simulink model "sm_bread_slicer"  (R2021b)
settings: Solver=ode15s  StartTime=0.0  StopTime=10  MaxStep=0.01  RelTol=1e-3  EnableMultiTasking=on
model workspace (MATLAB code in the model file):
  | lgrey = [0.6 0.6 0.6];
  | dgrey = [0.4 0.4 0.4];
  | blue = [0.0 0.6 1.0];
  | orange = [0.8 0.5 0.0];
  | dgreen = [0.0 0.3 0.0];
  | brown = [0.3 0.2 0.0];
  | red = [0.9 0.3 0.2];
  | yellow = [0.9 0.7 0.2];
  | rho_alum = 2700;
undefined symbols (not defined in the file): X, Y, Z
libraries: sm_lib x22, sm_bread_slicer_lib x10, fl_lib x8, nesl_utility x1
Description:
  | Rotational Interface : Electrically Operated Bread Slicer
  | 
  | This model simulates an electrically operated 1-DOF bread
  | slicing mechanism. The electrical motor circuit is modeled in
  | Simscape(TM) while the bread slicing mechanism is modeled
  | in Simscape Multibody(TM). The model uses a Revolute-Rotational
  | Interface block (blue block) to interface the electrical and 3D
  | mechanical parts of the model.
settings Model: Creator=The MathWorks, Inc.  LastModifiedBy=The MathWorks, Inc.
settings SolverCC: AlgebraicLoopSolver=TrustRegion
settings DataIOCC: LimitDataPoints=on  SaveFormat=Array  ReturnWorkspaceOutputs=off
settings OptimizationCC: ExpressionDepthLimit=2147483647  LifeSpan=inf
settings DebuggingCC: UnderspecifiedInitializationDetection=Classic  MergeDetectMultiDrivingBlocksExec=none  SolverPrmCheckMsg=warning  StateNameClashWarn=warning  SFUnexpectedBacktrackingDiag=warning  SFNoUnconditionalDefaultTransitionDiag=warning  SFExecutionAtInitializationDiag=none  SFMachineParentedDataDiag=warning  ArithmeticOperatorsInVariantConditions=warning
settings HardwareCC: ProdBitPerPointer=32  ProdBitPerSizeT=32  ProdBitPerPtrDiffT=32  ProdLargestAtomicFloat=None  ProdIntDivRoundTo=Undefined  ProdEndianess=Unspecified  ProdWordSize=32  ProdHWDeviceType=32-bit Generic
settings ModelReferenceCC: PropagateSignalLabelsOutOfModel=off
settings SFSimCC: SimUseLocalCustomCode=off  CustomCodeUndefinedFunction=UseInterfaceOnly
settings RTWCC: RTWUseLocalCustomCode=off
settings CodeAppCC: StateflowObjectComments=on
settings GRTTargetCC: TargetLangStandard=C89/C90 (ANSI)
settings ConfigComp: CovMetricSettings=dw  CovSaveCumulativeToWorkspaceVar=on  CovSaveSingleToWorkspaceVar=on  CovExternalEMLEnable=off  CovSFcnEnable=off
settings SimscapeCC: SimscapeNormalizeSystem=off  SimscapeLogType=all  SimscapeLogSimulationStatistics=on  SimscapeLogName=simlog_sm_bread_slicer
settings ConfigurationSet: Description=SimMechanics 2G
settings DiagnosticsConfigSet: SimMechanicsUnconnectedFramePorts=none
settings ExplorerConfigSet: InternalSimMechanicsExplorerSettings="<ExplorerConfiguration><canonicalview>default</canonicalview><TilePanel><TileInfo><Tiles Columns=\"1\" Count=\"1\" Rows=\"1\"><Column Left=\"2\" Weight=\"1\"/><Column Left=\"418\"/><Row Top=\"2\" Weight=\"1\"/><Row Top=\"419\"/><Tile Height=\"1\" Width=\"1\" X=\"0\" Y=\"0\"/></Tiles></TileInfo><SceneInfo><SceneViewer><BGColor><R>0.60000002384185791</R><G>0.60000002384185791</G><B>0.60000002384185791</B></BGColor><Camera><Position><X>0.97822830794307525</X><Y>-0.8448557030961209</Y><Z>0.99010983822795684</Z></Position><Center><X>0.13337260484695435</X><Y>0</Y><Z>0.14525413513183594</Z></Center><Up><X>-0.40824829046386307</X><Y>0.40824829046386307</Y><Z>0.81649658092772615</Z></Up><Left>-0.49494555294513704</Left><Right>0.49494555294513704</Right><Bottom>-0.45368637889623642</Bottom><Top>0.45368637889623642</Top></Camera></SceneViewer></SceneInfo></TilePanel></ExplorerConfiguration>"

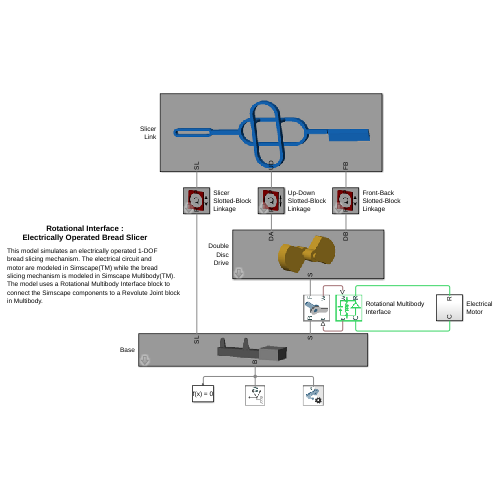
[thumbnail: Simulink's stored preview of the top-level diagram]
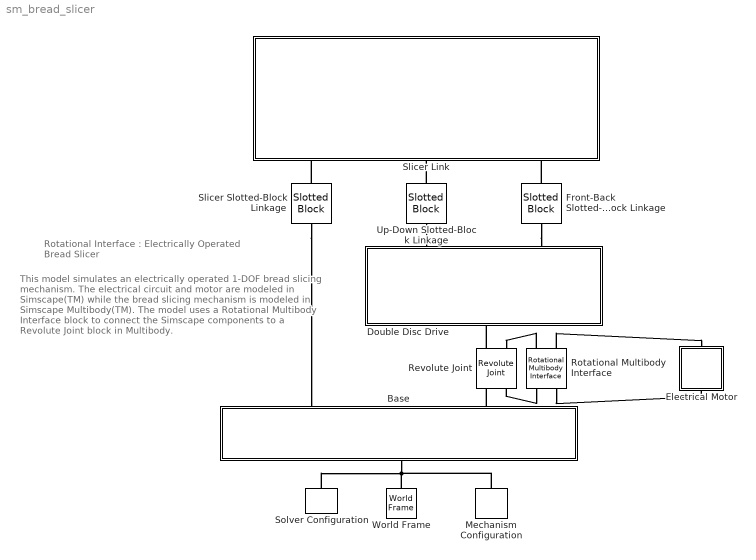
== system sm_bread_slicer ==
  note: This model simulates an electrically operated 1-DOF
      | bread slicing mechanism. The electrical circuit and
      | motor are modeled in Simscape(TM) while the bread
      | slicing mechanism is modeled in Simscape Multibody(TM).
      | The model uses a Rotational Multibody Interface block to
      | connect the Simscape components to a Revolute Joint block in Multibody.
  note: Rotational Interface :
      | Electrically Operated Bread Slicer
  Base : Subsystem  mask(Bread Slicer Base){L=70, W=15, H=10, Lct=30, Wct=30, Hct=14, Oha=-30, Ha=12, Wa=8, Ta=2, Rta=3, Rpa=0.75, Lpa=9, Hb=15, Wb=12, Tb=1.5, Rtb=3, clr=dgrey, rho=rho_alum}
      mask prompts: L "Base length (cm):"; W "Base width (cm):"; H "Base height (cm):"; Lct "Cutting table length (cm):"; Wct "Cutting table width (cm):"; Hct "Cutting table height (cm):"; Oha "Offset (cm):"; Ha "Height of hinge (cm):"; Wa "Base width of hinge (cm):"; Ta "Thickness of hinge (cm):"; Rta "Radius of curvature of top (cm):"; Rpa "Radius of pin:"; Lpa "Length of pin:"; Hb "Height of hinge (cm):"; Wb "Base width of hinge (cm):"; Tb "Thickness of hinge (cm):"; Rtb "Radius of curvature of top (cm):"; clr "Color:"; rho "Density (kg/m^3):"
      mask help: Base ground body on which the bread slicer mechanism is mounted on.
      mask Display:
      | image('sm_bread_slicer_base.png');
      | port_label('RConn',1,'SL');
      | port_label('RConn',2,'S');
      | port_label('LConn',1,'B');
  Double Disc Drive : Subsystem  mask(Double Disc Drive){R=5, T=4, Sa=150, S=6, Op=3, Rp=1, Lp=12, clr=yellow, rho=rho_alum}
      mask prompts: R "Disc radius (cm):"; T "Disc thickness (cm):"; Sa "Disc sector angle (deg):"; S "Disc separation (cm):"; Op "Pin offset (cm):"; Rp "Pin radius (cm):"; Lp "Pin length (cm):"; clr "Disc color [r g b]:"; rho "Density (kg/m^3):"
      mask help: Shaft with two rigidly attached opposing disc segments. The disc segments can fit and revolve within circular cavities. The port S refers to the shaft frame and must be attached to a revolute joint. The ports DA and DB refer to the frames at the center of the disc segments.
      mask init:
      | Sar = Sa*pi/180;
      | theta = linspace(-Sar/2,Sar/2,100)';
      | disc_xsec = [R*cos(theta) R*sin(theta)];
      | theta = linspace(Sar/2,2*pi-Sar/2,200)';
      | disc_xsec = [disc_xsec; 2*Rp*cos(theta)-Op 2*Rp*sin(theta)];
      mask Display:
      | image('sm_bread_slicer_drive.png');
      | port_label('RConn',1,'DA');
      | port_label('RConn',2,'DB');
      | port_label('LConn',1,'S');
  Electrical Motor : Subsystem
  Front-Back Slotted-Block Linkage : sm_bread_slicer_lib/Slotted Block  Lb=12  Wb=11  Tb=2  Rh=5  clr=red  rho=rho_alum
      settings: SourceProductBaseCode=MS
  Mechanism Configuration : sm_lib/Utilities/Mechanism Configuration  UniformGravity=Constant  GravityVector=[0 0 -9.81]  GravityUnits=m/s^2  LinearizationDelta=0.001  JointModeTransitionNonlinearIterations=2
  Revolute Joint : sm_lib/Joints/Revolute Joint  JointMode=Normal  SenseConstraintForce=off  SenseConstraintForceX=off  SenseConstraintForceY=off  SenseConstraintForceZ=off  SenseConstraintTorque=off  SenseConstraintTorqueX=off  SenseConstraintTorqueY=off  SenseConstraintTorqueZ=off  SenseTotalForce=off  SenseTotalForceX=off  SenseTotalForceY=off  SenseTotalForceZ=off  SenseTotalTorque=off  SenseTotalTorqueX=off  SenseTotalTorqueY=off  SenseTotalTorqueZ=off  CompositeWrenchDir=FollowerOnBase  CompositeWrenchFrame=BaseFrame  EquilibriumPosition=0  EquilibriumPositionUnits=deg  SpringStiffness=0  SpringStiffnessUnits=N*m/deg  DampingCoefficient=0  DampingCoefficientUnits=N*m/(deg/s)  TorqueActuationMode=InputTorque  MotionActuationMode=ComputedMotion  SensePosition=off  SenseVelocity=on  SenseAcceleration=off  SenseTorqueForce=off  SenseLowerLimitTorqueForce=off  SenseUpperLimitTorqueForce=off  LowerLimitSpecify=off  LowerLimitBound=-90  LowerLimitBoundUnits=deg  LowerLimitStiffness=1e4  LowerLimitStiffnessUnits=N*m/deg  LowerLimitDamping=10  LowerLimitDampingUnits=N*m/(deg/s)  LowerLimitTransitionRegionWidth=0.1  LowerLimitTransitionRegionWidthUnits=deg  UpperLimitSpecify=off  UpperLimitBound=90  UpperLimitBoundUnits=deg  UpperLimitStiffness=1e4  UpperLimitStiffnessUnits=N*m/deg  UpperLimitDamping=10  UpperLimitDampingUnits=N*m/(deg/s)  UpperLimitTransitionRegionWidth=0.1  UpperLimitTransitionRegionWidthUnits=deg  PositionTargetSpecify=on  PositionTargetPriority=Low  PositionTargetValue=90  PositionTargetValueUnits=deg  VelocityTargetSpecify=off  VelocityTargetPriority=High  VelocityTargetValue=0  VelocityTargetValueUnits=deg/s
  Rotational Multibody Interface : fl_lib/Mechanical/Multibody Interfaces/Rotational Multibody Interface
      settings: SourceProductBaseCode=SS
  Slicer Link : Subsystem  mask(Bread Slicer Link){}
      mask Display:
      | image('sm_bread_slicer_link.png');
      | port_label('LConn',1,'SL');
      | port_label('LConn',2,'UD');
      | port_label('LConn',3,'FB');
  Slicer Slotted-Block Linkage : sm_bread_slicer_lib/Slotted Block  Lb=4  Wb=2  Tb=2  Rh=0.75  clr=red  rho=rho_alum
      settings: SourceProductBaseCode=MS
  Solver Configuration : nesl_utility/Solver Configuration  PhysicalDomain=network_engine_domain  SubClassName=solver  LeftPortType=input  RightPortType=generic  Tones=[]  Harmonics=[]  SimulateNoise=off  Profile=off  UseLocalSampling=off  EnableSwitchedLinearOptims=on  FrequencyDomain=off  UseCCode=off  RelTol=0.001  AbsTol=1e-06  MinStep=1e-09  ToWorkspace=off  RevertToSquareIcSolve=off  NumHomotopyIterations=100  PhasorMode=off  PhasorModeNumHarmonics=1  DoDC=off  ResidualTolerance=1e-9  UseLocalSolver=off  LocalSolverChoice=NE_BACKWARD_EULER_ADVANCER  LocalSolverSampleTime=.001  DoFixedCost=off  MaxNonlinIter=3  MaxModeIter=2  ComputeImpulses=off  ImpulseIterations=2  LinearAlgebra=Sparse  EquationFormulation=NE_TIME_EF  DelaysMemoryBudget=1024  AutomaticFiltering=on  FilteringTimeConstant=0.001  PartitionStorageMethod=AS_NEEDED  PartitionMemoryBudget=1024  PartitionMethod=FAST
      settings: SourceProductBaseCode=PW,SS
  Up-Down Slotted-Block Linkage : sm_bread_slicer_lib/Slotted Block  Lb=12  Wb=11  Tb=2  Rh=5  clr=red  rho=rho_alum
      settings: SourceProductBaseCode=MS
  World Frame : sm_lib/Frames and Transforms/World Frame
  connections:
  World Frame/RConn1 -- Mechanism Configuration/RConn1 -- Solver Configuration/RConn1 -- Base/LConn1
  Slicer Slotted-Block Linkage/RConn1 -- Slicer Link/LConn1
  Slicer Slotted-Block Linkage/LConn1 -- Base/RConn1
  Up-Down Slotted-Block Linkage/RConn1 -- Slicer Link/LConn2
  Up-Down Slotted-Block Linkage/LConn1 -- Double Disc Drive/RConn1
  Front-Back Slotted-Block Linkage/RConn1 -- Slicer Link/LConn3
  Front-Back Slotted-Block Linkage/LConn1 -- Double Disc Drive/RConn2
  Revolute Joint/RConn1 -- Double Disc Drive/LConn1
  Rotational Multibody Interface/RConn1 -- Revolute Joint/RConn2
  Rotational Multibody Interface/LConn1 -- Revolute Joint/LConn2
  Base/RConn2 -- Revolute Joint/LConn1
  Rotational Multibody Interface/LConn2 -- Electrical Motor/LConn1
  Rotational Multibody Interface/RConn2 -- Electrical Motor/RConn1

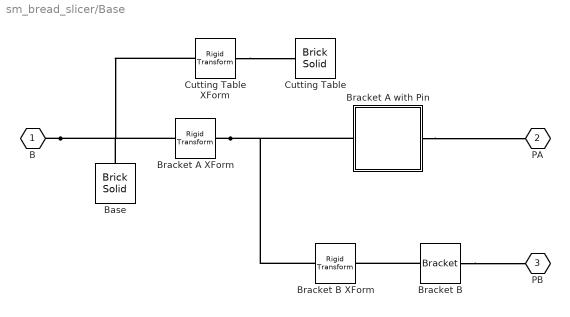
== system sm_bread_slicer/Base ==
  Base : sm_lib/Body Elements/Brick Solid  GraphicAmbientColor=[0.15 0.15 0.15 1.0]  BasedOnType=Density  BrickDimensions=[L W H]  BrickDimensionUnits=cm  CenterOfMass=[0 0 0]  CenterOfMassUnits=m  GraphicDiffuseColor=clr  Density=1000  DensityUnits=kg/(m^3)  DoExposeReferenceFrame=on  GraphicEmissiveColor=[0.0 0.0 0.0 1.0]  ExportEntireGeometry=off  SerializedFrames=<Frames/>  MarkerShape=Sphere  MarkerSize=10  GraphicType=FromGeometry  InertiaType=CalculateFromGeometry  Mass=1  MassUnits=kg  MomentsOfInertia=[1 1 1]  MomentsOfInertiaUnits=kg*m^2  GraphicOpacity=1.0  ProductsOfInertia=[0 0 0]  ProductsOfInertiaUnits=kg*m^2  GraphicShininess=75  GraphicSpecularColor=[0.5 0.5 0.5 1.0]  GraphicVisPropType=SimpleVisualProperties
  Bracket A XForm : sm_lib/Frames and Transforms/Rigid Transform  TranslationMethod=Cartesian  TranslationStandardOffset=0  TranslationLengthUnit=cm  TranslationStandardAxis=+Z  TranslationCartesianOffset=[Oha 0 H/2]  TranslationROffset=0  TranslationROffsetUnits=m  TranslationZOffset=0  TranslationZOffsetUnits=m  TranslationThetaOffset=0  TranslationThetaOffsetUnits=deg  RotationMethod=AlignedAxes  RotationAngleUnits=deg  RotationStandardAxis=+Z  RotationAngle=0  RotationArbitraryAxis=[0 0 1]  FollAlignAxisA=+Y  BaseAlignAxisA=+Z  FollAlignAxisB=+Z  BaseAlignAxisB=-Y  RotationSequenceAxes=FollowerAxes  RotationSequence=XYX  RotationSequenceAngles=[0 0 0]  RotationSequenceAnglesUnits=deg  RotationMatrix=[1 0 0; 0 1 0; 0 0 1]
  Bracket A with Pin : Subsystem  mask(Bracket with Pin){H=Ha, W=Wa, T=Ta, Rt=Rta, Rp=Rpa, Lp=Lpa, Oh=3, clr=clr, rho=rho}
      mask prompts: H "Height of hinge (cm):"; W "Base width of hinge (cm):"; T "Thickness of hinge (cm):"; Rt "Radius of curvature of top (cm):"; Rp "Pin radius (cm):"; Lp "Pin length (cm):"; Oh "Hinge point offset (cm)"; clr "Color:"; rho "Density:"
      mask init:
      | d = sqrt((H-Rt)^2 + (W/2)^2);
      | thd = acos(Rt/d) + acos((H-Rt)/d) - pi/2;
      | theta = linspace(thd,pi-thd,100)';
      | hinge_xsec = [W/2 0; Rt*cos(theta) (H-Rt)+Rt*sin(theta); -W/2 0];
  Bracket B : sm_bread_slicer_lib/Bracket  H=Hb  W=Wb  T=Tb  Rt=Rtb  clr=clr  rho=rho
      settings: SourceProductBaseCode=MS
  Bracket B XForm : sm_lib/Frames and Transforms/Rigid Transform  TranslationMethod=Cartesian  TranslationStandardOffset=39.5  TranslationLengthUnit=cm  TranslationStandardAxis=+X  TranslationCartesianOffset=[39.5 0 6]  TranslationROffset=0  TranslationROffsetUnits=m  TranslationZOffset=0  TranslationZOffsetUnits=m  TranslationThetaOffset=0  TranslationThetaOffsetUnits=deg  RotationMethod=None  RotationAngleUnits=deg  RotationStandardAxis=+Z  RotationAngle=90  RotationArbitraryAxis=[0 0 1]  FollAlignAxisA=+X  BaseAlignAxisA=+Y  FollAlignAxisB=+Y  BaseAlignAxisB=+Z  RotationSequenceAxes=FollowerAxes  RotationSequence=XYX  RotationSequenceAngles=[0 0 0]  RotationSequenceAnglesUnits=deg  RotationMatrix=[1 0 0; 0 1 0; 0 0 1]
  Cutting Table : sm_lib/Body Elements/Brick Solid  GraphicAmbientColor=[0.15 0.15 0.15 1.0]  BasedOnType=Density  BrickDimensions=[Lct Wct Hct]  BrickDimensionUnits=cm  CenterOfMass=[0 0 0]  CenterOfMassUnits=m  GraphicDiffuseColor=clr+0.2  Density=1000  DensityUnits=kg/(m^3)  DoExposeReferenceFrame=on  GraphicEmissiveColor=[0.0 0.0 0.0 1.0]  ExportEntireGeometry=off  SerializedFrames=<Frames/>  MarkerShape=Sphere  MarkerSize=10  GraphicType=FromGeometry  InertiaType=CalculateFromGeometry  Mass=1  MassUnits=kg  MomentsOfInertia=[1 1 1]  MomentsOfInertiaUnits=kg*m^2  GraphicOpacity=1.0  ProductsOfInertia=[0 0 0]  ProductsOfInertiaUnits=kg*m^2  GraphicShininess=75  GraphicSpecularColor=[0.5 0.5 0.5 1.0]  GraphicVisPropType=SimpleVisualProperties
  Cutting Table XForm : sm_lib/Frames and Transforms/Rigid Transform  TranslationMethod=Cartesian  TranslationStandardOffset=0  TranslationLengthUnit=cm  TranslationStandardAxis=+X  TranslationCartesianOffset=[L/2+Lct/2 0 (Hct-H)/2]  TranslationROffset=0  TranslationROffsetUnits=m  TranslationZOffset=0  TranslationZOffsetUnits=m  TranslationThetaOffset=0  TranslationThetaOffsetUnits=deg  RotationMethod=None  RotationAngleUnits=deg  RotationStandardAxis=+Z  RotationAngle=0  RotationArbitraryAxis=[0 0 1]  FollAlignAxisA=+Y  BaseAlignAxisA=+Z  FollAlignAxisB=+Z  BaseAlignAxisB=-Y  RotationSequenceAxes=FollowerAxes  RotationSequence=XYX  RotationSequenceAngles=[0 0 0]  RotationSequenceAnglesUnits=deg  RotationMatrix=[1 0 0; 0 1 0; 0 0 1]
  B : PMIOPort  Side=Left
  PA : PMIOPort  Port=2  Side=Right
  PB : PMIOPort  Port=3  Side=Right
  connections:
  B/RConn1 -- Base/RConn1 -- Cutting Table XForm/LConn1 -- Bracket A XForm/LConn1
  Bracket A XForm/RConn1 -- Bracket B XForm/LConn1 -- Bracket A with Pin/LConn1
  Bracket B/RConn1 -- PB/RConn1
  Cutting Table XForm/RConn1 -- Cutting Table/RConn1
  Bracket B/LConn1 -- Bracket B XForm/RConn1
  Bracket A with Pin/RConn1 -- PA/RConn1

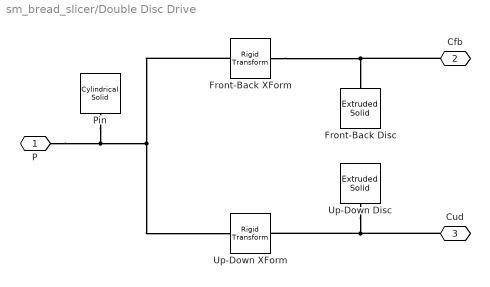
== system sm_bread_slicer/Double Disc Drive ==
  Front-Back Disc : sm_lib/Body Elements/Extruded Solid  GraphicAmbientColor=[0.15 0.15 0.15 1.0]  BasedOnType=Density  CenterOfMass=[0 0 0]  CenterOfMassUnits=m  GraphicDiffuseColor=clr  ExportConvexHullGeometry=off  ExtrusionCrossSection=disc_xsec  ExtrusionCrossSectionUnits=cm  Density=rho  DensityUnits=kg/(m^3)  DoExposeReferenceFrame=on  GraphicEmissiveColor=[0.0 0.0 0.0 1.0]  ExportEntireGeometry=off  ExtrusionLength=T  ExtrusionLengthUnits=cm  ExtrusionType=General  SerializedFrames=<Frames/>  MarkerShape=Sphere  MarkerSize=10  GraphicType=FromGeometry  InertiaType=CalculateFromGeometry  Mass=1  MassUnits=kg  MomentsOfInertia=[1 1 1]  MomentsOfInertiaUnits=kg*m^2  PolygonNumSides=3  GraphicOpacity=1.0  PolygonOuterRadius=1  PolygonOuterRadiusUnits=m  ProductsOfInertia=[0 0 0]  ProductsOfInertiaUnits=kg*m^2  GraphicShininess=75  GraphicSpecularColor=[0.5 0.5 0.5 1.0]  GraphicVisPropType=SimpleVisualProperties
  Front-Back XForm : sm_lib/Frames and Transforms/Rigid Transform  TranslationMethod=Cartesian  TranslationStandardOffset=0  TranslationLengthUnit=cm  TranslationStandardAxis=+Y  TranslationCartesianOffset=[-Op 0 -S/2]  TranslationROffset=0  TranslationROffsetUnits=m  TranslationZOffset=0  TranslationZOffsetUnits=m  TranslationThetaOffset=0  TranslationThetaOffsetUnits=deg  RotationMethod=AlignedAxes  RotationAngleUnits=deg  RotationStandardAxis=+Z  RotationAngle=90  RotationArbitraryAxis=[0 0 1]  FollAlignAxisA=+X  BaseAlignAxisA=-X  FollAlignAxisB=+Y  BaseAlignAxisB=-Y  RotationSequenceAxes=FollowerAxes  RotationSequence=XYX  RotationSequenceAngles=[0 0 0]  RotationSequenceAnglesUnits=deg  RotationMatrix=[1 0 0; 0 1 0; 0 0 1]
  Pin : sm_lib/Body Elements/Cylindrical Solid  GraphicAmbientColor=[0.15 0.15 0.15 1.0]  BasedOnType=Density  CenterOfMass=[0 0 0]  CenterOfMassUnits=m  GraphicDiffuseColor=clr  CylinderLength=Lp  CylinderLengthUnits=cm  CylinderRadius=Rp  CylinderRadiusUnits=cm  Density=rho  DensityUnits=kg/(m^3)  DoExposeReferenceFrame=on  GraphicEmissiveColor=[0.0 0.0 0.0 1.0]  ExportEntireGeometry=off  SerializedFrames=<Frames/>  MarkerShape=Sphere  MarkerSize=10  GraphicType=FromGeometry  InertiaType=CalculateFromGeometry  Mass=1  MassUnits=kg  MomentsOfInertia=[1 1 1]  MomentsOfInertiaUnits=kg*m^2  GraphicOpacity=1.0  ProductsOfInertia=[0 0 0]  ProductsOfInertiaUnits=kg*m^2  GraphicShininess=75  GraphicSpecularColor=[0.5 0.5 0.5 1.0]  GraphicVisPropType=SimpleVisualProperties
  Up-Down Disc : sm_lib/Body Elements/Extruded Solid  GraphicAmbientColor=[0.15 0.15 0.15 1.0]  BasedOnType=Density  CenterOfMass=[0 0 0]  CenterOfMassUnits=m  GraphicDiffuseColor=clr  ExportConvexHullGeometry=off  ExtrusionCrossSection=disc_xsec  ExtrusionCrossSectionUnits=cm  Density=rho  DensityUnits=kg/(m^3)  DoExposeReferenceFrame=on  GraphicEmissiveColor=[0.0 0.0 0.0 1.0]  ExportEntireGeometry=off  ExtrusionLength=T  ExtrusionLengthUnits=cm  ExtrusionType=General  SerializedFrames=<Frames/>  MarkerShape=Sphere  MarkerSize=10  GraphicType=FromGeometry  InertiaType=CalculateFromGeometry  Mass=1  MassUnits=kg  MomentsOfInertia=[1 1 1]  MomentsOfInertiaUnits=kg*m^2  PolygonNumSides=3  GraphicOpacity=1.0  PolygonOuterRadius=1  PolygonOuterRadiusUnits=m  ProductsOfInertia=[0 0 0]  ProductsOfInertiaUnits=kg*m^2  GraphicShininess=75  GraphicSpecularColor=[0.5 0.5 0.5 1.0]  GraphicVisPropType=SimpleVisualProperties
  Up-Down XForm : sm_lib/Frames and Transforms/Rigid Transform  TranslationMethod=Cartesian  TranslationStandardOffset=0  TranslationLengthUnit=cm  TranslationStandardAxis=-Y  TranslationCartesianOffset=[Op 0 S/2]  TranslationROffset=0  TranslationROffsetUnits=m  TranslationZOffset=0  TranslationZOffsetUnits=m  TranslationThetaOffset=0  TranslationThetaOffsetUnits=deg  RotationMethod=None  RotationAngleUnits=deg  RotationStandardAxis=+Z  RotationAngle=90  RotationArbitraryAxis=[0 0 1]  FollAlignAxisA=+X  BaseAlignAxisA=+Y  FollAlignAxisB=+Y  BaseAlignAxisB=-X  RotationSequenceAxes=FollowerAxes  RotationSequence=XYX  RotationSequenceAngles=[0 0 0]  RotationSequenceAnglesUnits=deg  RotationMatrix=[1 0 0; 0 1 0; 0 0 1]
  P : PMIOPort  Side=Left
  Cfb : PMIOPort  Port=2  Side=Right
  Cud : PMIOPort  Port=3  Side=Right
  connections:
  Up-Down Disc/RConn1 -- Cud/RConn1 -- Up-Down XForm/RConn1
  Pin/RConn1 -- P/RConn1 -- Front-Back XForm/LConn1 -- Up-Down XForm/LConn1
  Front-Back XForm/RConn1 -- Cfb/RConn1 -- Front-Back Disc/RConn1

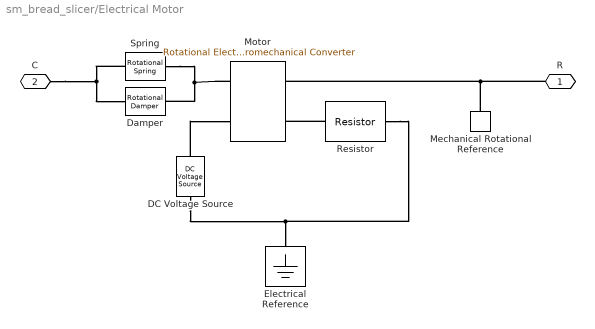
== system sm_bread_slicer/Electrical Motor ==
  DC Voltage Source : fl_lib/Electrical/Electrical Sources/DC Voltage Source  v0=50 V
  Damper : fl_lib/Mechanical/Rotational Elements/Rotational Damper  D=0.001 N*m/(rad/s)  w_specify=off  w_priority=High  w=0 rad/s  w_nominal_specify=off  w_nominal_unit=rad/s  w_nominal_value=1  t_specify=off  t_priority=High  t=0 N*m  t_nominal_specify=off  t_nominal_unit=N*m  t_nominal_value=1
  Electrical Reference : fl_lib/Electrical/Electrical Elements/Electrical Reference
  Mechanical Rotational Reference : fl_lib/Mechanical/Rotational Elements/Mechanical Rotational Reference
  Motor : fl_lib/Electrical/Electrical Elements/Rotational Electromechanical Converter  K=-5 V/(rad/s)  i_specify=off  i_priority=High  i=0 A  i_nominal_specify=off  i_nominal_unit=A  i_nominal_value=1  v_specify=off  v_priority=High  v=0 V  v_nominal_specify=off  v_nominal_unit=V  v_nominal_value=1  t_specify=off  t_priority=High  t=0 N*m  t_nominal_specify=off  t_nominal_unit=N*m  t_nominal_value=1  w_specify=off  w_priority=High  w=0 rad/s  w_nominal_specify=off  w_nominal_unit=rad/s  w_nominal_value=1
  Resistor : fl_lib/Electrical/Electrical Elements/Resistor  R=1 Ohm  i_specify=off  i_priority=High  i=0 A  i_nominal_specify=off  i_nominal_unit=A  i_nominal_value=1  v_specify=off  v_priority=High  v=0 V  v_nominal_specify=off  v_nominal_unit=V  v_nominal_value=1
  Spring : fl_lib/Mechanical/Rotational Elements/Rotational Spring  spr_rate=10 N*m/rad  w_specify=off  w_priority=High  w=0 rad/s  w_nominal_specify=off  w_nominal_unit=rad/s  w_nominal_value=1  t_specify=off  t_priority=High  t=0 N*m  t_nominal_specify=off  t_nominal_unit=N*m  t_nominal_value=1  phi_specify=on  phi_priority=High  phi=0 rad  phi_nominal_specify=off  phi_nominal_unit=rad  phi_nominal_value=1
  R : PMIOPort  Side=Right
  C : PMIOPort  Port=2  Side=Left
  connections:
  Spring/LConn1 -- C/RConn1 -- Damper/LConn1
  Spring/RConn1 -- Motor/LConn2 -- Damper/RConn1
  DC Voltage Source/LConn1 -- Motor/LConn1
  Resistor/LConn1 -- Motor/RConn1
  DC Voltage Source/RConn1 -- Electrical Reference/LConn1 -- Resistor/RConn1
  R/RConn1 -- Mechanical Rotational Reference/LConn1 -- Motor/RConn2

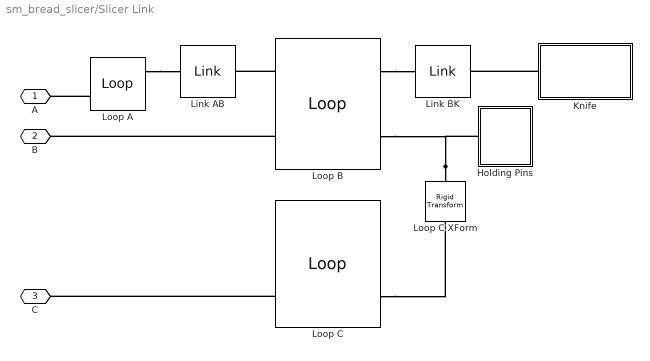
== system sm_bread_slicer/Slicer Link ==
  Holding Pins : Subsystem
  Knife : Subsystem  mask{L=20, W=6, Wb=2, Tb=0.5, clr=blue, rho=rho_alum}
      mask prompts: L "Length of knife (cm):"; W "Total width of knife (cm):"; Wb "Base width of knife (cm):"; Tb "Base thickness of knife (cm):"; clr "Color [r g b]:"; rho "Density (kg/m^3):"
      mask init:
      | knife_xsec = [0 -Tb/2; Wb -Tb/2; W 0; Wb Tb/2; 0 Tb/2];
      mask Display: image('sm_bread_slicer_knife.png');
  Link AB : sm_bread_slicer_lib/Link  L=11  W=2  T=2  Rl=2  Rr=7  clr=blue  rho=rho_alum
      settings: SourceProductBaseCode=MS
  Link BK : sm_bread_slicer_lib/Link  L=10  W=2  T=2  Rl=7  Rr=1000  clr=blue  rho=rho_alum
      settings: SourceProductBaseCode=MS
  Loop A : sm_bread_slicer_lib/Loop  L=15  W=4  T=2  Ws=2  clr=blue  rho=rho_alum
      settings: SourceProductBaseCode=MS
  Loop B : sm_bread_slicer_lib/Loop  L=25  W=14  T=2  Ws=11  clr=blue  rho=rho_alum
      settings: SourceProductBaseCode=MS
  Loop C : sm_bread_slicer_lib/Loop  L=25  W=14  T=2  Ws=11  clr=blue  rho=rho_alum
      settings: SourceProductBaseCode=MS
  Loop C XForm : sm_lib/Frames and Transforms/Rigid Transform  TranslationMethod=Cartesian  TranslationStandardOffset=6  TranslationLengthUnit=cm  TranslationStandardAxis=+Z  TranslationCartesianOffset=[0 0 6]  TranslationROffset=0  TranslationROffsetUnits=m  TranslationZOffset=0  TranslationZOffsetUnits=m  TranslationThetaOffset=0  TranslationThetaOffsetUnits=deg  RotationMethod=StandardAxis  RotationAngleUnits=deg  RotationStandardAxis=+Z  RotationAngle=90  RotationArbitraryAxis=[0 0 1]  FollAlignAxisA=+X  BaseAlignAxisA=+Y  FollAlignAxisB=+Y  BaseAlignAxisB=+Z  RotationSequenceAxes=FollowerAxes  RotationSequence=XYX  RotationSequenceAngles=[0 0 0]  RotationSequenceAnglesUnits=deg  RotationMatrix=[1 0 0; 0 1 0; 0 0 1]
  A : PMIOPort  Side=Left
  B : PMIOPort  Port=2  Side=Left
  C : PMIOPort  Port=3  Side=Left
  connections:
  Loop A/RConn1 -- Link AB/LConn1
  Loop A/LConn2 -- A/RConn1
  Loop B/LConn1 -- Link AB/RConn1
  Loop B/RConn1 -- Link BK/LConn1
  Loop C XForm/LConn1 -- Holding Pins/LConn1 -- Loop B/RConn2
  Loop C/RConn2 -- Loop C XForm/RConn1
  Loop C/LConn2 -- C/RConn1
  Loop B/LConn2 -- B/RConn1
  Knife/LConn1 -- Link BK/RConn1

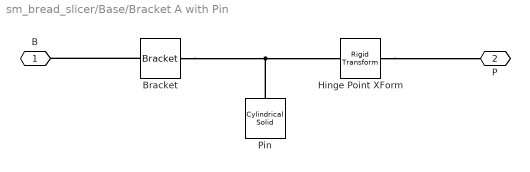
== system sm_bread_slicer/Base/Bracket A with Pin ==
  Bracket : sm_bread_slicer_lib/Bracket  H=H  W=W  T=T  Rt=Rt  clr=clr  rho=rho
      settings: SourceProductBaseCode=MS
  Hinge Point XForm : sm_lib/Frames and Transforms/Rigid Transform  TranslationMethod=Cartesian  TranslationStandardOffset=0  TranslationLengthUnit=cm  TranslationStandardAxis=+Y  TranslationCartesianOffset=[0 0 Oh]  TranslationROffset=0  TranslationROffsetUnits=m  TranslationZOffset=0  TranslationZOffsetUnits=m  TranslationThetaOffset=0  TranslationThetaOffsetUnits=deg  RotationMethod=None  RotationAngleUnits=deg  RotationStandardAxis=+Z  RotationAngle=0  RotationArbitraryAxis=[0 0 1]  FollAlignAxisA=+X  BaseAlignAxisA=+Y  FollAlignAxisB=+Y  BaseAlignAxisB=+Z  RotationSequenceAxes=FollowerAxes  RotationSequence=XYX  RotationSequenceAngles=[0 0 0]  RotationSequenceAnglesUnits=deg  RotationMatrix=[1 0 0; 0 1 0; 0 0 1]
  Pin : sm_lib/Body Elements/Cylindrical Solid  GraphicAmbientColor=[0.15 0.15 0.15 1.0]  BasedOnType=Density  CenterOfMass=[0 0 0]  CenterOfMassUnits=m  GraphicDiffuseColor=clr  CylinderLength=Lp  CylinderLengthUnits=cm  CylinderRadius=Rp  CylinderRadiusUnits=cm  Density=rho  DensityUnits=kg/(m^3)  DoExposeReferenceFrame=on  GraphicEmissiveColor=[0.0 0.0 0.0 1.0]  ExportEntireGeometry=off  SerializedFrames=<Frames/>  MarkerShape=Sphere  MarkerSize=10  GraphicType=FromGeometry  InertiaType=CalculateFromGeometry  Mass=1  MassUnits=kg  MomentsOfInertia=[1 1 1]  MomentsOfInertiaUnits=kg*m^2  GraphicOpacity=1.0  ProductsOfInertia=[0 0 0]  ProductsOfInertiaUnits=kg*m^2  GraphicShininess=75  GraphicSpecularColor=[0.5 0.5 0.5 1.0]  GraphicVisPropType=SimpleVisualProperties
  B : PMIOPort  Side=Left
  P : PMIOPort  Port=2  Side=Right
  connections:
  Pin/RConn1 -- Bracket/RConn1 -- Hinge Point XForm/LConn1
  Hinge Point XForm/RConn1 -- P/RConn1
  Bracket/LConn1 -- B/RConn1

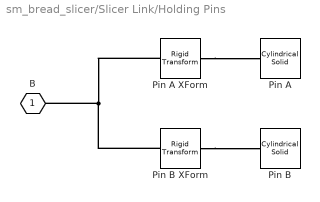
== system sm_bread_slicer/Slicer Link/Holding Pins ==
  Pin A : sm_lib/Body Elements/Cylindrical Solid  GraphicAmbientColor=[0.15 0.15 0.15 1.0]  BasedOnType=Density  CenterOfMass=[0 0 0]  CenterOfMassUnits=m  GraphicDiffuseColor=blue  CylinderLength=4  CylinderLengthUnits=cm  CylinderRadius=1  CylinderRadiusUnits=cm  Density=rho_alum  DensityUnits=kg/(m^3)  DoExposeReferenceFrame=on  GraphicEmissiveColor=[0.0 0.0 0.0 1.0]  ExportEntireGeometry=off  SerializedFrames=<Frames/>  MarkerShape=Sphere  MarkerSize=10  GraphicType=FromGeometry  InertiaType=CalculateFromGeometry  Mass=1  MassUnits=kg  MomentsOfInertia=[1 1 1]  MomentsOfInertiaUnits=kg*m^2  GraphicOpacity=1.0  ProductsOfInertia=[0 0 0]  ProductsOfInertiaUnits=kg*m^2  GraphicShininess=75  GraphicSpecularColor=[0.5 0.5 0.5 1.0]  GraphicVisPropType=SimpleVisualProperties
  Pin A XForm : sm_lib/Frames and Transforms/Rigid Transform  TranslationMethod=Cartesian  TranslationStandardOffset=6  TranslationLengthUnit=cm  TranslationStandardAxis=+Z  TranslationCartesianOffset=[-6.25 6.25 3]  TranslationROffset=0  TranslationROffsetUnits=m  TranslationZOffset=0  TranslationZOffsetUnits=m  TranslationThetaOffset=0  TranslationThetaOffsetUnits=deg  RotationMethod=None  RotationAngleUnits=deg  RotationStandardAxis=+Z  RotationAngle=90  RotationArbitraryAxis=[0 0 1]  FollAlignAxisA=+X  BaseAlignAxisA=+Y  FollAlignAxisB=+Y  BaseAlignAxisB=+Z  RotationSequenceAxes=FollowerAxes  RotationSequence=XYX  RotationSequenceAngles=[0 0 0]  RotationSequenceAnglesUnits=deg  RotationMatrix=[1 0 0; 0 1 0; 0 0 1]
  Pin B : sm_lib/Body Elements/Cylindrical Solid  GraphicAmbientColor=[0.15 0.15 0.15 1.0]  BasedOnType=Density  CenterOfMass=[0 0 0]  CenterOfMassUnits=m  GraphicDiffuseColor=blue  CylinderLength=4  CylinderLengthUnits=cm  CylinderRadius=1  CylinderRadiusUnits=cm  Density=rho_alum  DensityUnits=kg/(m^3)  DoExposeReferenceFrame=on  GraphicEmissiveColor=[0.0 0.0 0.0 1.0]  ExportEntireGeometry=off  SerializedFrames=<Frames/>  MarkerShape=Sphere  MarkerSize=10  GraphicType=FromGeometry  InertiaType=CalculateFromGeometry  Mass=1  MassUnits=kg  MomentsOfInertia=[1 1 1]  MomentsOfInertiaUnits=kg*m^2  GraphicOpacity=1.0  ProductsOfInertia=[0 0 0]  ProductsOfInertiaUnits=kg*m^2  GraphicShininess=75  GraphicSpecularColor=[0.5 0.5 0.5 1.0]  GraphicVisPropType=SimpleVisualProperties
  Pin B XForm : sm_lib/Frames and Transforms/Rigid Transform  TranslationMethod=Cartesian  TranslationStandardOffset=6  TranslationLengthUnit=cm  TranslationStandardAxis=+Z  TranslationCartesianOffset=[6.25 6.25 3]  TranslationROffset=0  TranslationROffsetUnits=m  TranslationZOffset=0  TranslationZOffsetUnits=m  TranslationThetaOffset=0  TranslationThetaOffsetUnits=deg  RotationMethod=None  RotationAngleUnits=deg  RotationStandardAxis=+Z  RotationAngle=90  RotationArbitraryAxis=[0 0 1]  FollAlignAxisA=+X  BaseAlignAxisA=+Y  FollAlignAxisB=+Y  BaseAlignAxisB=+Z  RotationSequenceAxes=FollowerAxes  RotationSequence=XYX  RotationSequenceAngles=[0 0 0]  RotationSequenceAnglesUnits=deg  RotationMatrix=[1 0 0; 0 1 0; 0 0 1]
  B : PMIOPort  Side=Left
  connections:
  Pin B XForm/RConn1 -- Pin B/RConn1
  Pin A XForm/RConn1 -- Pin A/RConn1
  Pin A XForm/LConn1 -- Pin B XForm/LConn1 -- B/RConn1

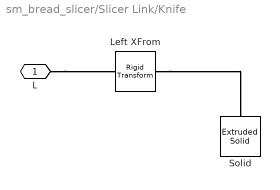
== system sm_bread_slicer/Slicer Link/Knife ==
  Left XFrom : sm_lib/Frames and Transforms/Rigid Transform  TranslationMethod=Cartesian  TranslationStandardOffset=L/2  TranslationLengthUnit=cm  TranslationStandardAxis=-Z  TranslationCartesianOffset=[Wb/2 0 -L/2]  TranslationROffset=0  TranslationROffsetUnits=m  TranslationZOffset=0  TranslationZOffsetUnits=m  TranslationThetaOffset=0  TranslationThetaOffsetUnits=deg  RotationMethod=AlignedAxes  RotationAngleUnits=deg  RotationStandardAxis=+Z  RotationAngle=0  RotationArbitraryAxis=[0 0 1]  FollAlignAxisA=+X  BaseAlignAxisA=+Z  FollAlignAxisB=+Z  BaseAlignAxisB=-Y  RotationSequenceAxes=FollowerAxes  RotationSequence=XYX  RotationSequenceAngles=[0 0 0]  RotationSequenceAnglesUnits=deg  RotationMatrix=[1 0 0; 0 1 0; 0 0 1]
  Solid : sm_lib/Body Elements/Extruded Solid  GraphicAmbientColor=[0.15 0.15 0.15 1.0]  BasedOnType=Density  CenterOfMass=[0 0 0]  CenterOfMassUnits=m  GraphicDiffuseColor=clr  ExportConvexHullGeometry=off  ExtrusionCrossSection=knife_xsec  ExtrusionCrossSectionUnits=cm  Density=rho  DensityUnits=kg/(m^3)  DoExposeReferenceFrame=on  GraphicEmissiveColor=[0.0 0.0 0.0 1.0]  ExportEntireGeometry=off  ExtrusionLength=L  ExtrusionLengthUnits=cm  ExtrusionType=General  SerializedFrames=<Frames/>  MarkerShape=Sphere  MarkerSize=10  GraphicType=FromGeometry  InertiaType=CalculateFromGeometry  Mass=1  MassUnits=kg  MomentsOfInertia=[1 1 1]  MomentsOfInertiaUnits=kg*m^2  PolygonNumSides=3  GraphicOpacity=1.0  PolygonOuterRadius=1  PolygonOuterRadiusUnits=m  ProductsOfInertia=[0 0 0]  ProductsOfInertiaUnits=kg*m^2  GraphicShininess=75  GraphicSpecularColor=[0.5 0.5 0.5 1.0]  GraphicVisPropType=SimpleVisualProperties
  L : PMIOPort  Side=Left
  connections:
  L/RConn1 -- Left XFrom/RConn1
  Left XFrom/LConn1 -- Solid/RConn1
